simulink model "RosTest_R2018b"  (R2018b)
settings: Solver=VariableStepAuto  StartTime=0.0  StopTime=inf  RelTol=1e-3
libraries: robotlib x1
settings Model: Creator=51078  LastModifiedBy=51078

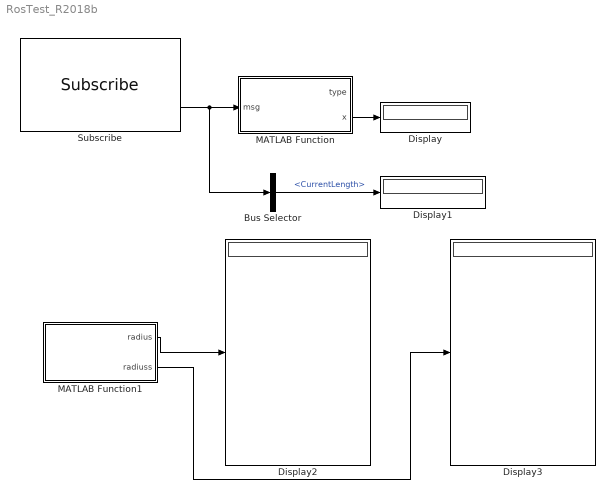
== system RosTest_R2018b ==
  Bus Selector : BusSelector  OutputSignals=Units_SL_Info.CurrentLength
  Display{,1..3} (4 alike) : Display
  MATLAB Function : MATLAB Function  TreatAsAtomicUnit=on
  MATLAB Function1 : MATLAB Function
  Subscribe : robotlib/Subscribe  topicSource=Select from ROS network  topic=/decision_info  messageType=swarm_msgs/Pipeline  sampleTime=-1  messageQueueLength=1
  wires:
  Subscribe/2 -> Bus Selector/1, MATLAB Function/1(msg)
  MATLAB Function/2(x) -> Display/1
  Bus Selector/1 -> Display1/1  "<CurrentLength>"
  MATLAB Function1/1(radius) -> Display2/1
  MATLAB Function1/2(radiuss) -> Display3/1

== matlab function RosTest_R2018b/MATLAB Function1 ==
  data: radius output; radiuss output
function [radius,radiuss]   = fcn
coder.extrinsic('csape')
EncirclePoint=[113,1.7;161,-9;211,-5;248,-18;262,-6;260,13;252,27;202,29;132,23;116,16;113,1.7];
EncirclePoint_x=EncirclePoint(:,1);
EncirclePoint_y=EncirclePoint(:,2);
k=length(EncirclePoint_x);
xx=csape(1:k,EncirclePoint_x,'periodic');
yy=csape(1:k,EncirclePoint_y,'periodic');
curve_x=ppval(xx,linspace(1,k,100*k));
curve_y=ppval(yy,linspace(1,k,100*k));

radius=zeros(100*k,2);
for i=1:length(radius(:,1))
    radius(i,1)=curve_x(i);
    radius(i,2)=curve_y(i);
end

k=1:length(EncirclePoint_x);
ki=linspace(1,length(EncirclePoint_x),1000); %%%%% 插值的点越多，控制更精确，曲线更光滑，计算更耗时
curve_xx=(interp1(k,EncirclePoint_x,ki,'linear'))';
curve_yy=(interp1(k,EncirclePoint_y,ki,'linear'))';
radiuss=zeros(1000,2);
for i=1:length(radiuss(:,1))
    radiuss(i,1)=curve_xx(i);
    radiuss(i,2)=curve_yy(i);
end

== matlab function RosTest_R2018b/MATLAB Function ==
  data: type output; msg input; x output
function [type,x] = fcn(msg)
type = msg.Pipetype.Data;
x = msg.Units(17).Right.X;
